simulink model "host_model"  (R2019a)
settings: Solver=FixedStepAuto  StartTime=0.0  StopTime=inf  FixedStep=1/30  RelTol=1e-3  EnableMultiTasking=on
PreLoadFcn:
  | load('visionhdlLaneDetectionInit.mat');
  | 
  | %Birds-Eye View Parameters:
  | T_unreal = [-0.346719845290643,-3.45626583672944e-16,-2.42608110520569e-19;-1.76272742794994,-2.62399506819665,-0.00185184300876343;1283.14845282490,1569.57420684550,1];
  | shiftleft = single([-5,-5,-5,-5,-5,-5,-5,-5,-5,-5,   -5,-4,-2,-2,-2,-2,0,0,0,1,    1,2,3,4,5,6,7,10,11,13,     15,17,20,22,26,30,33,38,42,46]);
  | shiftright = single([-20,-20,-20,-20,-20,-20,-20,-20,-20,-20,    -20,-20,-20,-21,-22,-23,-24,-24,-24,-25,    -26,-27,-28,-29,-30,-32,-33,-35,-37,-39,    -41,-45,-46,-50,-53,-57,-61,-67,-72,-78]);
libraries: visiontextngfix x2, xpcutilitieslib x1, dspvision x1, simulink x1, xpcrtudplib x1, visionsinks x1
settings Model: EnablePacing=on  Creator=speedgoat  LastModifiedBy=timo.straessle
settings SolverCC: ConcurrentTasks=on  AutoInsertRateTranBlk=on
settings DataIOCC: SaveFormat=StructureWithTime
settings OptimizationCC: BlockReduction=off  OptimizeBlockIOStorage=off  BufferReuse=off  GlobalBufferReuse=off  ExpressionFolding=off  LocalBlockOutputs=off  OptimizeDataStoreBuffers=off  BusAssignmentInplaceUpdate=off
settings HardwareCC: ProdBitPerPointer=32  ProdBitPerSizeT=32  ProdBitPerPtrDiffT=32  ProdLargestAtomicFloat=None  ProdWordSize=32  ProdLongLongMode=on  ProdHWDeviceType=Generic->32-bit x86 compatible
settings RTWCC: SystemTargetFile=slrt.tlc  TemplateMakefile=slrt_default_tmf  Description=Simulink Real-Time  CodeExecutionProfiling=on  RTWCompilerOptimization=on
settings SimulinkRealTimeCC: SupportVariableSizeSignals=on  PreserveStateflowLocalDataDimensions=off  RL32LogTETModifier=off  xPCConcurrentTasks=on

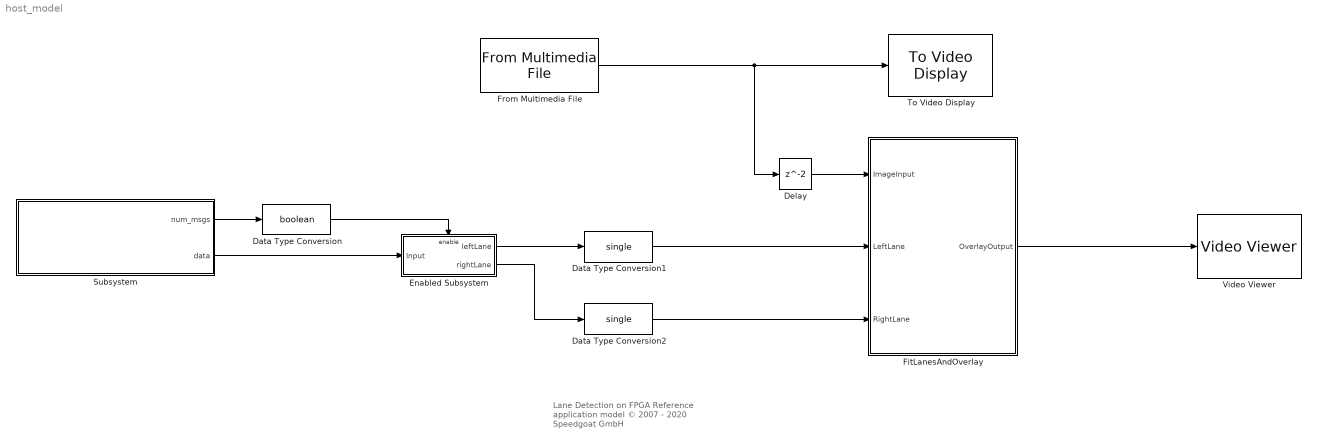
== system host_model ==
  note: Lane Detection on FPGA
      |
      | Reference application model
      | © 2007 - 2020 Speedgoat GmbH
  Data Type Conversion : DataTypeConversion  OutDataTypeStr=boolean
  Data Type Conversion1 : DataTypeConversion  OutDataTypeStr=single
  Data Type Conversion2 : DataTypeConversion  OutDataTypeStr=single
  Delay : Delay
  Enabled Subsystem : Subsystem  TreatAsAtomicUnit=on
  FitLanesAndOverlay : Subsystem
  From Multimedia File : dspvision/From Multimedia File  inputFilename=unreal.mp4  readRange=[1 Inf]  loop=on  numPlays=inf  outputStreams=Video only  videoDataType=uint8  audioDataType=double  inheritSampleTime=off  userDefinedSampleTime=1/30  noAudioOutput=off  isIntensityVideo=off  fourcc=RGB  colorVideoFormat=One multidimensional signal  outputEOF=off  dataOrg=Column-major  audioFrameSize=1024  computeAudioFrameSize=off  outSamplingMode=Sample based
      settings: SourceProductName=DSP System Toolbox  SourceProductBaseCode=DS
  Subsystem : Subsystem
  To Video Display : visionsinks/To Video Display  windowSizeMode=Full-screen (Esc to exit)  openAtMdlStart=on  fullScreen=off  videoWindowX=3440  videoWindowY=23  saveWindowSize=off  videoWindowWidth=1920  videoWindowHeight=1017  inputColorFormat=RGB  inputType=Obsolete  imagePorts=One multidimensional signal  OutputDevice=On-screen video monitor  dataOrg=Column-major  isWindowOpen=off
      settings: SourceProductName=Computer Vision Toolbox
  Video Viewer : VideoViewer  FigPos=[1 1398 3440 1298]
  wires:
  Data Type Conversion/1 -> Enabled Subsystem/Enable
  Subsystem/2(data) -> Enabled Subsystem/1(Input)
  Subsystem/1(num_msgs) -> Data Type Conversion/1
  Enabled Subsystem/1(leftLane) -> Data Type Conversion1/1
  Enabled Subsystem/2("rightLane ") -> Data Type Conversion2/1
  Data Type Conversion1/1 -> FitLanesAndOverlay/2(LeftLane)
  Data Type Conversion2/1 -> FitLanesAndOverlay/3(RightLane)
  From Multimedia File/1 -> Delay/1, To Video Display/1
  FitLanesAndOverlay/1(OverlayOutput) -> Video Viewer/1
  Delay/1 -> FitLanesAndOverlay/1(ImageInput)

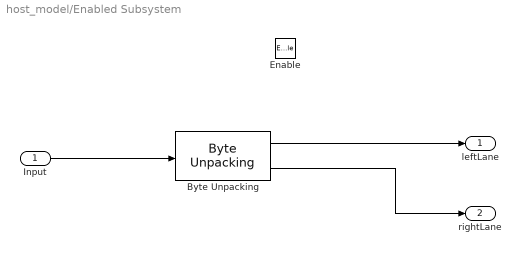
== system host_model/Enabled Subsystem ==
  Input : Inport
  Enable : EnablePort
  "Byte Unpacking " : xpcutilitieslib/Byte Unpacking   MaskUnpackedDataTypes={['uint16'],['uint16']}  MaskUnpackedDataSizes={[40],[40]}  MaskAlignment=1
      settings: SourceProductName=Simulink Real-Time  SourceProductBaseCode=XP
  leftLane : Outport
  "rightLane " : Outport  Port=2
  wires:
  "Byte Unpacking "/2 -> "rightLane "/1
  "Byte Unpacking "/1 -> leftLane/1
  Input/1 -> "Byte Unpacking "/1

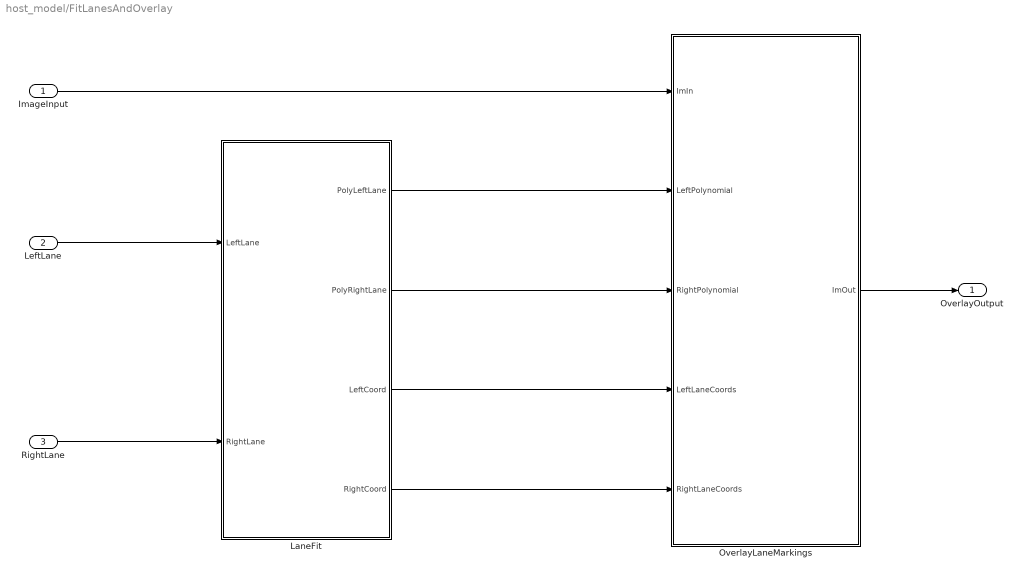
== system host_model/FitLanesAndOverlay ==
  ImageInput : Inport
  LeftLane : Inport  Port=2
  RightLane : Inport  Port=3
  LaneFit : Subsystem
  OverlayLaneMarkings : Subsystem
  OverlayOutput : Outport
  wires:
  OverlayLaneMarkings/1(ImOut) -> OverlayOutput/1
  LaneFit/1(PolyLeftLane) -> OverlayLaneMarkings/2(LeftPolynomial)
  LaneFit/4(RightCoord) -> OverlayLaneMarkings/5(RightLaneCoords)
  LaneFit/3(LeftCoord) -> OverlayLaneMarkings/4(LeftLaneCoords)
  LaneFit/2(PolyRightLane) -> OverlayLaneMarkings/3(RightPolynomial)
  ImageInput/1 -> OverlayLaneMarkings/1(ImIn)
  LeftLane/1 -> LaneFit/1(LeftLane)
  RightLane/1 -> LaneFit/2(RightLane)

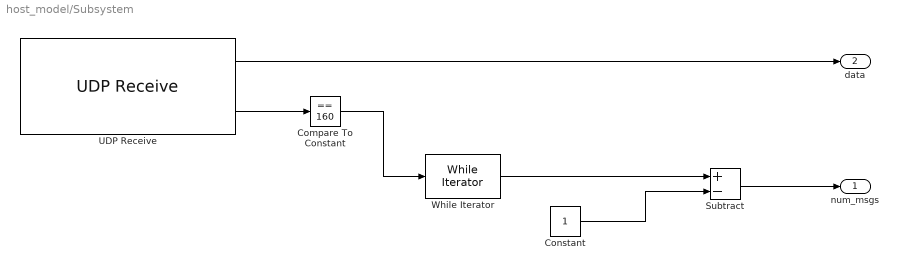
== system host_model/Subsystem ==
  Compare To Constant : simulink/Logic and Bit Operations/Compare To Constant  relop===  const=160  OutDataTypeStr=boolean
  Constant : Constant
  Subtract : Sum  Inputs=+-
  UDP Receive : xpcrtudplib/UDP Receive  ipAddressVal=Use host-target connection  localPort=8001  rcvWidth=160  rcvFmAny=off  fmAddress=192.168.7.1  rcvMulticast=off  multicastAddress={}  maxUDPQueue=8  sampleTime=-1
      settings: SourceProductName=Simulink Real-Time
  While Iterator : WhileIterator  WhileBlockType=do-while  ShowIterationPort=on
  num_msgs : Outport
  data : Outport  Port=2
  wires:
  UDP Receive/1 -> data/1
  UDP Receive/2 -> Compare To Constant/1
  Compare To Constant/1 -> While Iterator/1
  While Iterator/1 -> Subtract/1
  Constant/1 -> Subtract/2
  Subtract/1 -> num_msgs/1

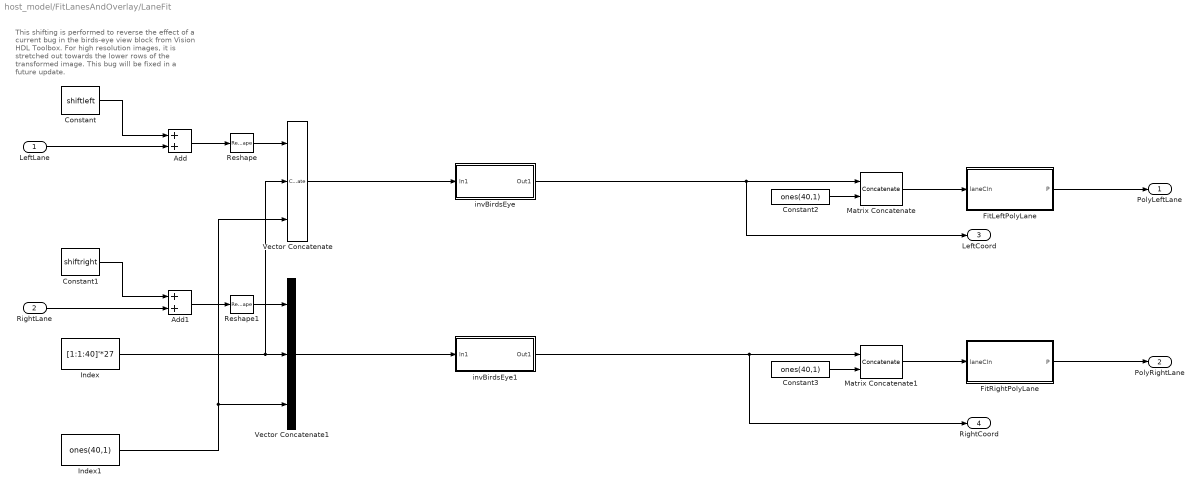
== system host_model/FitLanesAndOverlay/LaneFit ==
  note: This shifting is performed to reverse the effect of a current bug in the birds-eye view block from Vision HDL Toolbox. For high resolution images, it is stretched out towards the lower rows of the transformed image. This bug will be fixed in a future update.
  LeftLane : Inport
  RightLane : Inport  Port=2
  Add : Sum
  Add1 : Sum
  Constant : Constant  Value=shiftleft
  Constant1 : Constant  Value=shiftright
  Constant2 : Constant  Value=ones(40,1)  OutDataTypeStr=single
  Constant3 : Constant  Value=ones(40,1)  OutDataTypeStr=single
  FitLeftPolyLane : MATLAB Function  TreatAsAtomicUnit=on
  FitRightPolyLane : MATLAB Function  TreatAsAtomicUnit=on
  Index : Constant  Value=[1:1:40]'*27  VectorParams1D=off  OutDataTypeStr=single  SampleTime=-1
  Index1 : Constant  Value=ones(40,1)  VectorParams1D=off  OutDataTypeStr=single  SampleTime=-1
  Matrix Concatenate : Concatenate  Mode=Multidimensional array  ConcatenateDimension=2
  Matrix Concatenate1 : Concatenate  Mode=Multidimensional array  ConcatenateDimension=2
  Reshape : Reshape  OutputDimensionality=Column vector (2-D)
  Reshape1 : Reshape  OutputDimensionality=Column vector (2-D)
  Vector Concatenate : Concatenate  NumInputs=3  Mode=Multidimensional array  ConcatenateDimension=2
  Vector Concatenate1 : Concatenate  NumInputs=3  Mode=Multidimensional array  ConcatenateDimension=2
  invBirdsEye : Subsystem
  invBirdsEye1 : Subsystem
  PolyLeftLane : Outport
  PolyRightLane : Outport  Port=2
  LeftCoord : Outport  Port=3
  RightCoord : Outport  Port=4
  wires:
  FitLeftPolyLane/1(P) -> PolyLeftLane/1
  Vector Concatenate/1 -> invBirdsEye/1(In1)
  Index/1 -> Vector Concatenate/2, Vector Concatenate1/2
  Vector Concatenate1/1 -> invBirdsEye1/1(In1)
  FitRightPolyLane/1(P) -> PolyRightLane/1
  LeftLane/1 -> Add/2
  RightLane/1 -> Add1/2
  Constant/1 -> Add/1
  Add/1 -> Reshape/1
  Constant1/1 -> Add1/1
  Add1/1 -> Reshape1/1
  Index1/1 -> Vector Concatenate1/3, Vector Concatenate/3
  invBirdsEye/1(Out1) -> Matrix Concatenate/1, LeftCoord/1
  Reshape/1 -> Vector Concatenate/1
  Reshape1/1 -> Vector Concatenate1/1
  Constant2/1 -> Matrix Concatenate/2
  Matrix Concatenate/1 -> FitLeftPolyLane/1(laneCIn)
  invBirdsEye1/1(Out1) -> Matrix Concatenate1/1, RightCoord/1
  Constant3/1 -> Matrix Concatenate1/2
  Matrix Concatenate1/1 -> FitRightPolyLane/1(laneCIn)

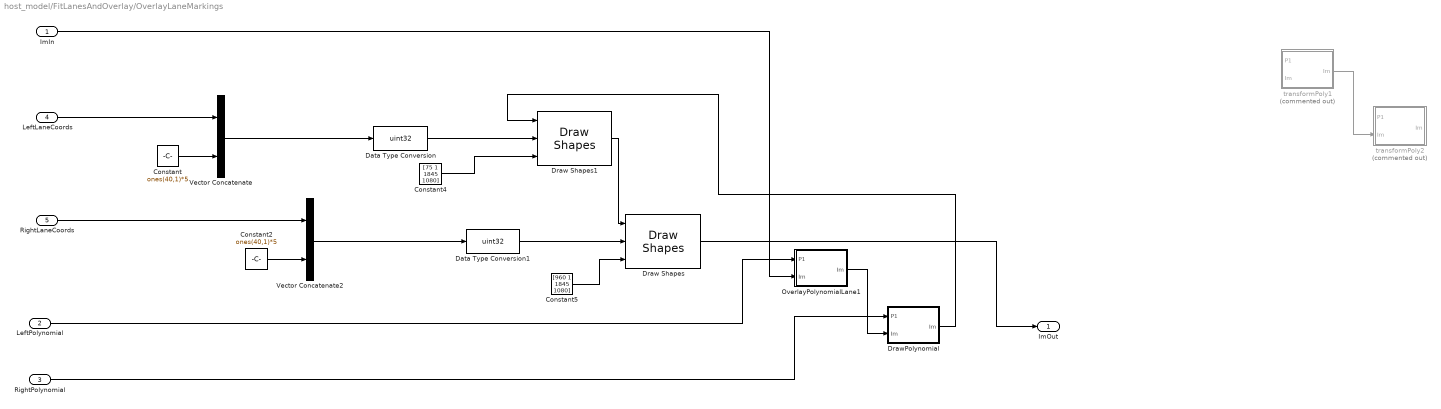
== system host_model/FitLanesAndOverlay/OverlayLaneMarkings ==
  ImIn : Inport
  LeftPolynomial : Inport  Port=2
  RightPolynomial : Inport  Port=3
  LeftLaneCoords : Inport  Port=4
  RightLaneCoords : Inport  Port=5
  Constant : Constant  Value=ones(40,1)*5  OutDataTypeStr=single  SampleTime=-1
  Constant2 : Constant  Value=ones(40,1)*5  OutDataTypeStr=single  SampleTime=-1
  Constant4 : Constant  Value=[75 1 1845 1080]  OutDataTypeStr=uint32  SampleTime=-1
  Constant5 : Constant  Value=[960 1 1845 1080]  OutDataTypeStr=uint32  SampleTime=-1
  Data Type Conversion : DataTypeConversion  OutDataTypeStr=uint32
  Data Type Conversion1 : DataTypeConversion  OutDataTypeStr=uint32
  Draw Shapes : visiontextngfix/Draw Shapes  shape=Circles  fill=off  lineWidth=3  fillClrSource=Specify via dialog  display=User-specified value  intensity=200  color=[10, 10, 255]  opacity=0.6  viewport=Specify region of interest via port  antialiasing=off  inType=Obsolete  imagePorts=One multidimensional signal  roundingMode=Floor  overflowMode=off  memoryMode=Specify word length  memoryWordLength=16  prodOutputMode=Binary point scaling  prodOutputWordLength=32  prodOutputFracLength=14  prodOutputSlope=2^-14  accumSlope=2^-14  memoryFracLength=15
      settings: SourceProductName=Computer Vision Toolbox
  Draw Shapes1 : visiontextngfix/Draw Shapes  shape=Circles  fill=off  lineWidth=3  fillClrSource=Specify via dialog  display=User-specified value  intensity=200  color=[10, 255, 10]  opacity=0.6  viewport=Specify region of interest via port  antialiasing=off  inType=Obsolete  imagePorts=One multidimensional signal  roundingMode=Floor  overflowMode=off  memoryMode=Specify word length  memoryWordLength=16  prodOutputMode=Binary point scaling  prodOutputWordLength=32  prodOutputFracLength=14  prodOutputSlope=2^-14  accumSlope=2^-14  memoryFracLength=15
      settings: SourceProductName=Computer Vision Toolbox
  DrawPolynomial : MATLAB Function  TreatAsAtomicUnit=on
  OverlayPolynomialLane1 : MATLAB Function  TreatAsAtomicUnit=on
  Vector Concatenate : Concatenate  Mode=Multidimensional array  ConcatenateDimension=2
  Vector Concatenate2 : Concatenate  Mode=Multidimensional array  ConcatenateDimension=2
  transformPoly1 : MATLAB Function  Commented=on  TreatAsAtomicUnit=on
  transformPoly2 : MATLAB Function  Commented=on  TreatAsAtomicUnit=on
  ImOut : Outport
  wires:
  RightLaneCoords/1 -> Vector Concatenate2/1
  Vector Concatenate/1 -> Data Type Conversion/1
  Constant/1 -> Vector Concatenate/2
  LeftLaneCoords/1 -> Vector Concatenate/1
  LeftPolynomial/1 -> OverlayPolynomialLane1/1(P1)
  Vector Concatenate2/1 -> Data Type Conversion1/1
  Constant4/1 -> Draw Shapes1/3
  RightPolynomial/1 -> DrawPolynomial/1(P1)
  Data Type Conversion1/1 -> Draw Shapes/2
  Draw Shapes1/1 -> Draw Shapes/1
  Constant5/1 -> Draw Shapes/3
  Data Type Conversion/1 -> Draw Shapes1/2
  Constant2/1 -> Vector Concatenate2/2
  OverlayPolynomialLane1/1(Im) -> DrawPolynomial/2("Im ")
  transformPoly1/1(Im) -> transformPoly2/2("Im ")
  ImIn/1 -> OverlayPolynomialLane1/2("Im ")
  DrawPolynomial/1(Im) -> Draw Shapes1/1
  Draw Shapes/1 -> ImOut/1

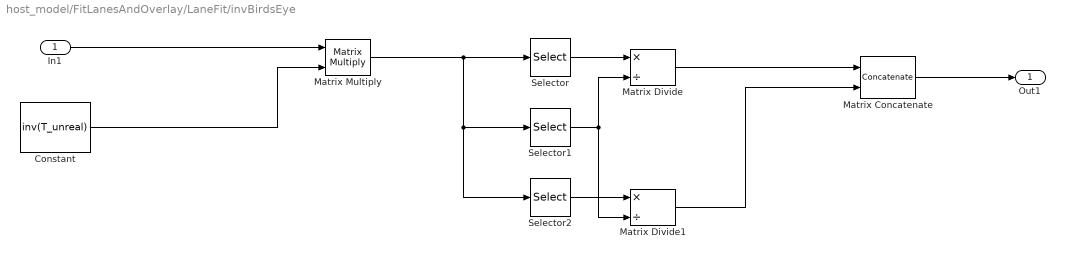
== system host_model/FitLanesAndOverlay/LaneFit/invBirdsEye ==
  In1 : Inport
  Constant : Constant  Value=inv(T_unreal)  OutDataTypeStr=single
  Matrix Concatenate : Concatenate  Mode=Multidimensional array  ConcatenateDimension=2
  Matrix Divide : Product  Inputs=*/
  Matrix Divide1 : Product  Inputs=*/
  Matrix Multiply : Product  Multiplication=Matrix(*)
  Selector : Selector  NumberOfDimensions=2  InputPortWidth=3  IndexOptions=Index vector (dialog),Index vector (dialog)  Indices=[1:40],[1]  OutputSizes=1,1
  Selector1 : Selector  NumberOfDimensions=2  InputPortWidth=3  IndexOptions=Index vector (dialog),Index vector (dialog)  Indices=[1:40],[3]  OutputSizes=1,1
  Selector2 : Selector  NumberOfDimensions=2  InputPortWidth=3  IndexOptions=Index vector (dialog),Index vector (dialog)  Indices=[1:40],[2]  OutputSizes=1,1
  Out1 : Outport
  wires:
  Constant/1 -> Matrix Multiply/2
  In1/1 -> Matrix Multiply/1
  Selector/1 -> Matrix Divide/1
  Selector1/1 -> Matrix Divide1/2, Matrix Divide/2
  Matrix Divide/1 -> Matrix Concatenate/1
  Selector2/1 -> Matrix Divide1/1
  Matrix Multiply/1 -> Selector/1, Selector2/1, Selector1/1
  Matrix Divide1/1 -> Matrix Concatenate/2
  Matrix Concatenate/1 -> Out1/1

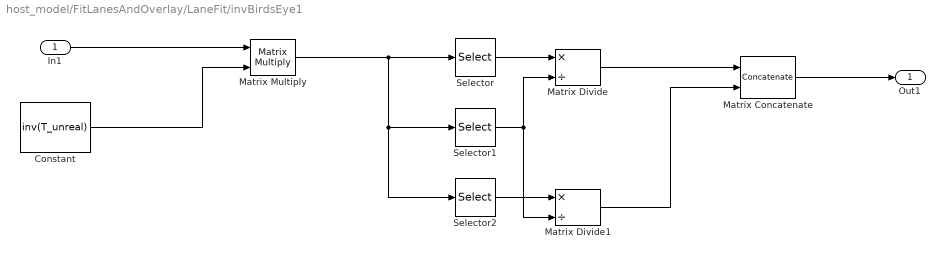
== system host_model/FitLanesAndOverlay/LaneFit/invBirdsEye1 ==
  In1 : Inport
  Constant : Constant  Value=inv(T_unreal)  OutDataTypeStr=single
  Matrix Concatenate : Concatenate  Mode=Multidimensional array  ConcatenateDimension=2
  Matrix Divide : Product  Inputs=*/
  Matrix Divide1 : Product  Inputs=*/
  Matrix Multiply : Product  Multiplication=Matrix(*)
  Selector : Selector  NumberOfDimensions=2  InputPortWidth=3  IndexOptions=Index vector (dialog),Index vector (dialog)  Indices=[1:40],[1]  OutputSizes=1,1
  Selector1 : Selector  NumberOfDimensions=2  InputPortWidth=3  IndexOptions=Index vector (dialog),Index vector (dialog)  Indices=[1:40],[3]  OutputSizes=1,1
  Selector2 : Selector  NumberOfDimensions=2  InputPortWidth=3  IndexOptions=Index vector (dialog),Index vector (dialog)  Indices=[1:40],[2]  OutputSizes=1,1
  Out1 : Outport
  wires:
  Matrix Concatenate/1 -> Out1/1
  Matrix Divide1/1 -> Matrix Concatenate/2
  Matrix Multiply/1 -> Selector1/1, Selector2/1, Selector/1
  Selector2/1 -> Matrix Divide1/1
  Matrix Divide/1 -> Matrix Concatenate/1
  Selector1/1 -> Matrix Divide/2, Matrix Divide1/2
  Selector/1 -> Matrix Divide/1
  In1/1 -> Matrix Multiply/1
  Constant/1 -> Matrix Multiply/2

== matlab function host_model/FitLanesAndOverlay/LaneFit/FitLeftPolyLane ==
  data: laneCIn input; P output
function P  = fitLane(laneCIn)

%#codegen

persistent P1;
if isempty(P1)
    P1 = [0 0 0];
end

T_unreal = [-0.346719845290643,-3.45626583672944e-16,-2.42608110520569e-19;-1.76272742794994,-2.62399506819665,-0.00185184300876343;1283.14845282490,1569.57420684550,1];
leftLimit = 50;

bev_pts = laneCIn*T_unreal;
bev_pts = bev_pts(:,1)./bev_pts(:,3);

% laneC = zeros(40,2);
inliersMask = zeros(1,100);
inlierTable1 = zeros(2,100);
P1T= single([0 0 0]);
% % aviod using sortrows (time complexity O(nlogn))
% % now O(n) oeprations
laneC = single(zeros(40,2));
 numG = 0;
 for jj = 1:1:40
     if(bev_pts(jj,1)>leftLimit)
         numG = numG+1;
         laneC(numG,1:2) = single(laneCIn(jj,1:2));
     end
 end


% ignore when inliers/total < curInliersRatio
curInliersRatio = 0.4;

% inlierIndex1-1 = num of inliers in best model
% is also used to determine whether a best model is found
inlierIndex1 = 0;

% K = log(1-P)/log(1-w^s)
K = 70; % max iteration

distanceMax = 960; % distance Threshold

curvatureMax = 0.003; % curvature Threshold for P(1); maybe removed for curved lanes


if numG>3
    
    %%% Use RANSAC for robust fit of 2nd order polynomial
    
    for ii = 1:1:K

        a = randperm(numG,3);
        
        P1T = polyfit(laneC(a,1), laneC(a,1),2);
        
        % O(n) operations
        numInliers = 0;
        for jj = 1:1:numG
            x1 = floor(polyval(P1T,laneC(jj,1)));
            inliersMask(jj) = abs(x1-laneC(jj,1))<distanceMax;
            if(inliersMask(jj))
                numInliers = numInliers + 1;
            end
        end

        if ((numInliers/numG)>curInliersRatio && abs(P1T(1))<curvatureMax && numInliers>2)
            % record the inliers for current best model  
            curInliersRatio = numInliers/numG;
            inlierIndex1 = 1;
            for jj = 1:1:numG
                if(inliersMask(jj))
                    inlierTable1(1,inlierIndex1) = laneC(jj,2);
                    inlierTable1(2,inlierIndex1) = laneC(jj,1);
                    inlierIndex1 = inlierIndex1 + 1;
                end
            end
        end
        
    end
  
end

    P1T = polyfit(inlierTable1(1,1:inlierIndex1-1), inlierTable1(2,1:inlierIndex1-1),2);


if abs(P1T(1))<curvatureMax % if found a best model; initial inlierIndex1 = 0;
    % refine the fitted line using all inliers
    P1 = P1T;
end

P = P1;

== matlab function host_model/FitLanesAndOverlay/LaneFit/FitRightPolyLane ==
  data: laneCIn input; P output
function P  = fitLane(laneCIn)

%#codegen

persistent P1;
if isempty(P1)
    P1 = [0 0 0];
end

T_unreal = [-0.346719845290643,-3.45626583672944e-16,-2.42608110520569e-19;-1.76272742794994,-2.62399506819665,-0.00185184300876343;1283.14845282490,1569.57420684550,1];
leftLimit = 50;

bev_pts = laneCIn*T_unreal;
bev_pts = bev_pts(:,1)./bev_pts(:,3);

% laneC = zeros(40,2);
inliersMask = zeros(1,100);
inlierTable1 = zeros(2,100);
P1T= single([0 0 0]);
% % aviod using sortrows (time complexity O(nlogn))
% % now O(n) oeprations
laneC = single(zeros(40,2));
 numG = 0;
 for jj = 1:1:40
     if(bev_pts(jj,1)>leftLimit)
         numG = numG+1;
         laneC(numG,1:2) = single(laneCIn(jj,1:2));
     end
 end


% ignore when inliers/total < curInliersRatio
curInliersRatio = 0.4;

% inlierIndex1-1 = num of inliers in best model
% is also used to determine whether a best model is found
inlierIndex1 = 0;

% K = log(1-P)/log(1-w^s)
K = 70; % max iteration

distanceMax = 960; % distance Threshold

curvatureMax = 0.003; % curvature Threshold for P(1); maybe removed for curved lanes


if numG>3
    
    %%% Use RANSAC for robust fit of 2nd order polynomial
    
    for ii = 1:1:K

        a = randperm(numG,3);
        
        P1T = polyfit(laneC(a,1), laneC(a,1),2);
        
        % O(n) operations
        numInliers = 0;
        for jj = 1:1:numG
            x1 = floor(polyval(P1T,laneC(jj,1)));
            inliersMask(jj) = abs(x1-laneC(jj,1))<distanceMax;
            if(inliersMask(jj))
                numInliers = numInliers + 1;
            end
        end

        if ((numInliers/numG)>curInliersRatio && abs(P1T(1))<curvatureMax && numInliers>2)
            % record the inliers for current best model  
            curInliersRatio = numInliers/numG;
            inlierIndex1 = 1;
            for jj = 1:1:numG
                if(inliersMask(jj))
                    inlierTable1(1,inlierIndex1) = laneC(jj,2);
                    inlierTable1(2,inlierIndex1) = laneC(jj,1);
                    inlierIndex1 = inlierIndex1 + 1;
                end
            end
        end
        
    end
  
end

    P1T = polyfit(inlierTable1(1,1:inlierIndex1-1), inlierTable1(2,1:inlierIndex1-1),2);


if abs(P1T(1))<curvatureMax % if found a best model; initial inlierIndex1 = 0;
    % refine the fitted line using all inliers
    P1 = P1T;
end

P = P1;

== matlab function host_model/FitLanesAndOverlay/OverlayLaneMarkings/DrawPolynomial ==
  data: P1 input; Im output; Im input
function Im  = DrawLane(P1,Im)
%#codegen

% ipmImage = uint8(zeros(900,640,3));
% HD: uint8(zeros(1575,1440,3));
RGBVal = [255,10,10];



  for ii = 580:1:830
      x1E = floor(polyval(P1,ii));
      
      if x1E <=5 || isnan(x1E)
          x1E = 6;
      elseif x1E>=1916
          x1E=1916;
      end
      
      Im(ii,x1E+4,:) = RGBVal;
      Im(ii,x1E+3,:) = RGBVal;
      Im(ii,x1E+2,:) = RGBVal;
      Im(ii,x1E+1,:) = RGBVal;
      Im(ii,x1E+0,:) = RGBVal;
      Im(ii,x1E-1,:) = RGBVal;
      Im(ii,x1E-2,:) = RGBVal;
      Im(ii,x1E-3,:) = RGBVal;
      Im(ii,x1E-4,:) = RGBVal;

      
  end


% Im = ipmImage;

== matlab function host_model/FitLanesAndOverlay/OverlayLaneMarkings/OverlayPolynomialLane1 ==
  data: P1 input; Im output; Im input
function Im  = fcn(P1,Im)
%#codegen

% ipmImage = uint8(zeros(900,640,3));
% HD: uint8(zeros(1575,1440,3));
RGBVal = [255,10,10];



  for ii = 580:1:830
      x1E = floor(polyval(P1,ii));
      
      if x1E <=50 || isnan(x1E)
          x1E = 6;
      elseif x1E>=1916
          x1E=1916;
      end
      
      Im(ii,x1E+4,:) = RGBVal;
      Im(ii,x1E+3,:) = RGBVal;
      Im(ii,x1E+2,:) = RGBVal;
      Im(ii,x1E+1,:) = RGBVal;
      Im(ii,x1E+0,:) = RGBVal;
      Im(ii,x1E-1,:) = RGBVal;
      Im(ii,x1E-2,:) = RGBVal;
      Im(ii,x1E-3,:) = RGBVal;
      Im(ii,x1E-4,:) = RGBVal;

      
  end


% Im = ipmImage;

== matlab function host_model/FitLanesAndOverlay/OverlayLaneMarkings/transformPoly2 ==
  data: P1 input; Im output; Im input
function Im  = DrawLane(P1,Im)
%#codegen

% ipmImage = uint8(zeros(900,640,3));
% HD: uint8(zeros(1575,1440,3));
RGBVal = [0,255,9];

T = [-2.90029596744358,2.68571999949696e-15,2.90693131678693e-18;12.3092646220043,6.97845044093522,0.0128996468512238;-13759.7104434929,-9905.42281289439,-17.3101474001826];

  for ii = 1:1:1575
      x1E = polyval(P1,ii);
      
      warped = floor([ii,x1E,1]*T);
      
      if 1<=warped(1) && warped(1)<=1080 && 6<=warped(2) && warped(2)<=1920
          Im(warped(1),warped(2)+0,:) = RGBVal;
          Im(warped(1),warped(2)-1,:) = RGBVal;
          Im(warped(1),warped(2)-2,:) = RGBVal;
          Im(warped(1),warped(2)-3,:) = RGBVal;
          Im(warped(1),warped(2)-4,:) = RGBVal;
          Im(warped(1),warped(2)-5,:) = RGBVal;
      end
  end
  
  end


% Im = ipmImage;

== matlab function host_model/FitLanesAndOverlay/OverlayLaneMarkings/transformPoly1 ==
  data: P1 input; Im output; Im input
function Im  = DrawLane(P1,Im)
%#codegen

% ipmImage = uint8(zeros(900,640,3));
% HD: uint8(zeros(1575,1440,3));
RGBVal = [0,255,9];

T = [-2.90029596744358,2.68571999949696e-15,2.90693131678693e-18;12.3092646220043,6.97845044093522,0.0128996468512238;-13759.7104434929,-9905.42281289439,-17.3101474001826];

  for ii = 1:1:1575
      x1E = polyval(P1,ii);
      
      warped = floor([ii,x1E,1]*T);
      
      if 1<=warped(1) && warped(1)<=1080 && 6<=warped(2) && warped(2)<=1920
          Im(warped(1),warped(2)+0,:) = RGBVal;
          Im(warped(1),warped(2)-1,:) = RGBVal;
          Im(warped(1),warped(2)-2,:) = RGBVal;
          Im(warped(1),warped(2)-3,:) = RGBVal;
          Im(warped(1),warped(2)-4,:) = RGBVal;
          Im(warped(1),warped(2)-5,:) = RGBVal;
      end
  end
  
  end


% Im = ipmImage;
